simulink model "Sim_NL_YZ"  (R2016a)
settings: Solver=ode45  StartTime=0.0  StopTime=2  RelTol=1e-3
settings Model: Creator=Florian  LastModifiedBy=Florian

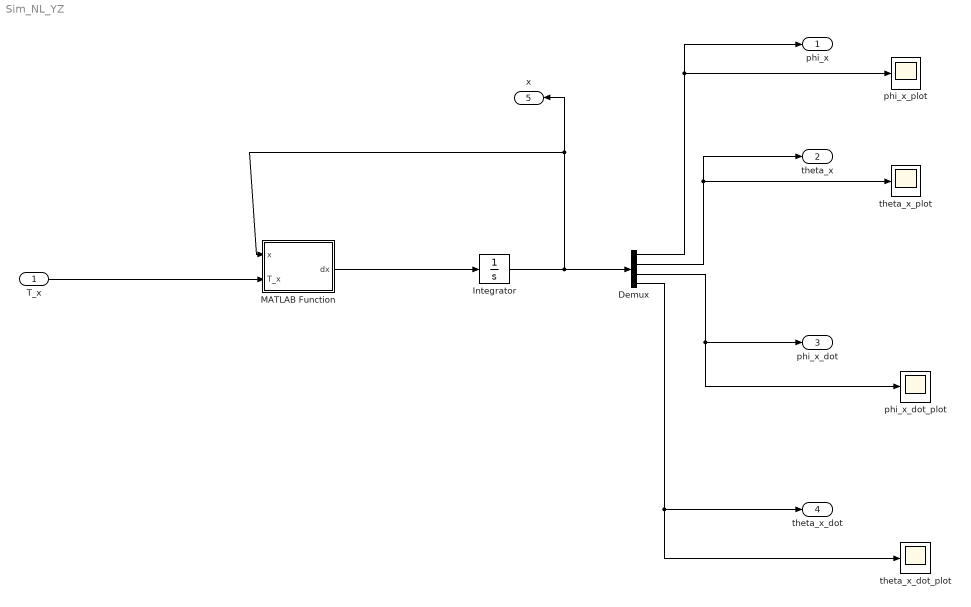
== system Sim_NL_YZ ==
  "T_x " : Inport
  Demux : Demux
  Integrator : Integrator  InitialCondition=[0 0 0 0]
  MATLAB Function : MATLAB Function  TreatAsAtomicUnit=on
  phi_x_dot_plot : Scope
  phi_x_plot : Scope
  theta_x_dot_plot : Scope
  theta_x_plot : Scope
  phi_x : Outport
  theta_x : Outport  Port=2
  phi_x_dot : Outport  Port=3
  theta_x_dot : Outport  Port=4
  x : Outport  Port=5
  wires:
  MATLAB Function/1(dx) -> Integrator/1
  Integrator/1 -> x/1, MATLAB Function/1(x), Demux/1
  Demux/1 -> phi_x_plot/1, phi_x/1
  Demux/2 -> theta_x/1, theta_x_plot/1
  Demux/3 -> phi_x_dot_plot/1, phi_x_dot/1
  Demux/4 -> theta_x_dot_plot/1, theta_x_dot/1
  "T_x "/1 -> MATLAB Function/2(T_x)

== matlab function Sim_NL_YZ/MATLAB Function ==
  data: x input; T_x input; dx output
function dx = fcn(x,T_x)

%Zuweisung Koordinaten und Ableitungen
phi_x =x(1);
theta_x=x(2);
phi_x_dot=x(3);
theta_x_dot=x(4);

phi_x_dotdot=(18014398509481984*(1474780203060832382832000000*sin(theta_x)*theta_x_dot^2 + 6673461925215283943359375000*T_x + 295268271287815685091301875*sin(theta_x) - 8944396862587810826384572416*cos(theta_x)*sin(theta_x) + 517041384719804006400000000*T_x*cos(theta_x)))/(75*(1807366736725976544289483038067261440000*cos(theta_x) - 27374775655728371289468879137739903074304*cos(theta_x)^2 + 200948944860727701207841270280447671484375));

theta_x_dotdot= -(9007199254740992*(22102728721212020468750000*T_x - 405980752992200943301368000*sin(theta_x) - 300987024758221901214375*theta_x_dot^2*sin(theta_x) + 41363310777584320512000000*T_x*cos(theta_x) + 9117631868081356601819136*theta_x_dot^2*cos(theta_x)*sin(theta_x)))/(3*(1807366736725976544289483038067261440000*cos(theta_x) - 27374775655728371289468879137739903074304*cos(theta_x)^2 + 200948944860727701207841270280447671484375));

%Zuweisung Ausgang
dx = [phi_x_dot; theta_x_dot; phi_x_dotdot; theta_x_dotdot];
end
